simulink model "Problem13_model"  (R2020a)
settings: Solver=ode4  StartTime=0.0  StopTime=SIM_TIME  RelTol=1e-3
values from neighbouring files (symbols this model uses):
  f1 = @(q3) (1/2*K4*q3^2 - 1/2*m3*L3*q3)    [Problem7_9.m]    (also in problem12.m = kT * K_D ./ Jeff; problem13.m = kT * K_D ./ Jeff; problem15.m = kT * K_p; problem18.m = kT * K_p)
  f2 = @(q3) (m4*a4*q3)    [Problem7_9.m]    (also in problem12.m = kT * K_p ./ Jeff; problem13.m = kT * K_p ./ Jeff; problem15.m = kT * K_D; problem18.m = kT * K_D)
  G = 1/n ./ Jeff    [problem13.m]    (also in problem15.m = tf([1/n^2, 0],1); problem18.m = tf([1/n^2, 0],1))
  n1 = (feff + kT * K_D)./Jeff    [problem12.m]    (also in problem13.m; problem15.m = kT*K_p; problem18.m = kT*K_p)
  n2 = kT * K_p ./ Jeff    [problem12.m]    (also in problem13.m; problem15.m = feff + kT*K_D; problem18.m = feff + kT*K_D)
  qr = [0.34, 0.34, 0.34, 0.34]    [problem12.m]    (also in problem13.m = [0.35, 0.35, 0.35, 0.35]; problem15.m = [0.35, 0.35, 0.35, 0.35]; problem16.m = [0.35, 0.35, 0.35, 0.35]; problem17.m = simout.qr)
  STEP_SIZE = 0.1    [Problem8_script.m]    (also in problem12.m = 0.01; problem13.m = 0.01; problem15.m = 0.001; problem16.m = 0.001)
  step_time = 0.01    [problem12.m]    (also in problem13.m; problem15.m; problem16.m)
  T_L = -abs(h)    [problem13.m]    (also in problem15.m = zeros(4,1); problem16.m = zeros(4,1); problem17.m = abs(h); problem18.m = abs(h))
settings Model: Creator=Theis  LastModifiedBy=Theis

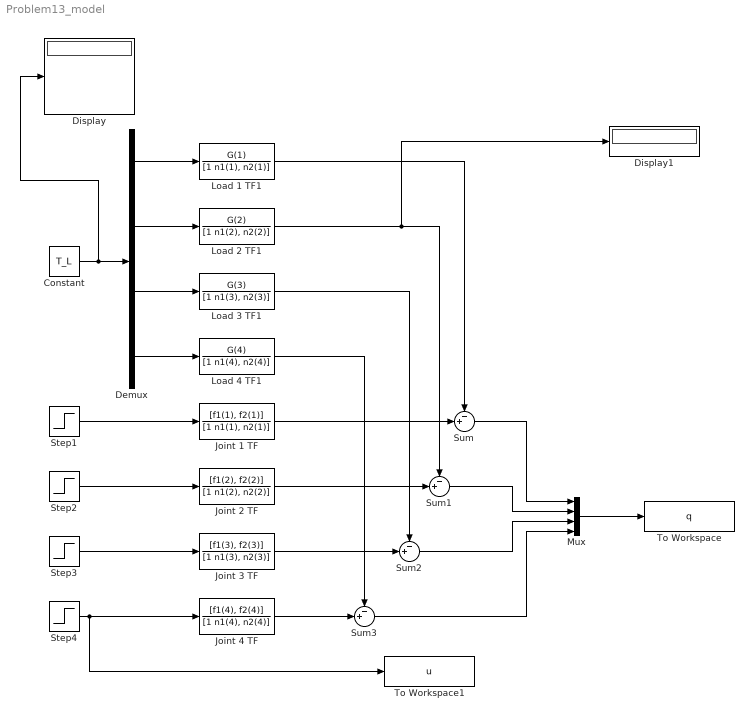
== system Problem13_model ==
  Constant : Constant  Value=T_L
  Demux : Demux
  Display : Display
  Display1 : Display
  Joint 1 TF : TransferFcn  Numerator=[f1(1), f2(1)]  Denominator=[1 n1(1), n2(1)]
  Joint 2 TF : TransferFcn  Numerator=[f1(2), f2(2)]  Denominator=[1 n1(2), n2(2)]
  Joint 3 TF : TransferFcn  Numerator=[f1(3), f2(3)]  Denominator=[1 n1(3), n2(3)]
  Joint 4 TF : TransferFcn  Numerator=[f1(4), f2(4)]  Denominator=[1 n1(4), n2(4)]
  Load 1 TF1 : TransferFcn  Numerator=G(1)  Denominator=[1 n1(1), n2(1)]
  Load 2 TF1 : TransferFcn  Numerator=G(2)  Denominator=[1 n1(2), n2(2)]
  Load 3 TF1 : TransferFcn  Numerator=G(3)  Denominator=[1 n1(3), n2(3)]
  Load 4 TF1 : TransferFcn  Numerator=G(4)  Denominator=[1 n1(4), n2(4)]
  Mux : Mux
  Step1 : Step  Time=step_time  After=qr(1)  SampleTime=0
  Step2 : Step  Time=step_time  After=qr(2)  SampleTime=0
  Step3 : Step  Time=step_time  After=qr(3)  SampleTime=0
  Step4 : Step  Time=step_time  After=qr(4)  SampleTime=0
  Sum{,1..3} (4 alike) : Sum  Inputs=-+|
  To Workspace : ToWorkspace  VariableName=q  SaveFormat=Timeseries  SampleTime=STEP_SIZE
  To Workspace1 : ToWorkspace  VariableName=u  SaveFormat=Timeseries  SampleTime=STEP_SIZE
  wires:
  Mux/1 -> To Workspace/1
  Sum/1 -> Mux/1
  Sum1/1 -> Mux/2
  Sum2/1 -> Mux/3
  Sum3/1 -> Mux/4
  Step3/1 -> Joint 3 TF/1
  Step2/1 -> Joint 2 TF/1
  Step1/1 -> Joint 1 TF/1
  Step4/1 -> Joint 4 TF/1, To Workspace1/1
  Constant/1 -> Display/1, Demux/1
  Joint 1 TF/1 -> Sum/2
  Joint 2 TF/1 -> Sum1/2
  Joint 3 TF/1 -> Sum2/2
  Joint 4 TF/1 -> Sum3/2
  Demux/1 -> Load 1 TF1/1
  Demux/2 -> Load 2 TF1/1
  Demux/3 -> Load 3 TF1/1
  Demux/4 -> Load 4 TF1/1
  Load 4 TF1/1 -> Sum3/1
  Load 3 TF1/1 -> Sum2/1
  Load 2 TF1/1 -> Display1/1, Sum1/1
  Load 1 TF1/1 -> Sum/1
